simulink model "pdl_nonlinear_hw1"  (R2017a)
settings: Solver=VariableStepAuto  StartTime=0.0  StopTime=duration  RelTol=1e-3
values from neighbouring files (symbols this model uses):
  b = 0.1    [pendulum_hw1.m]
  f_p = 0    [pendulum_hw1.m]
  g = 9.81    [pendulum_hw1.m]
  k = 0.15    [pendulum_hw1.m]
  L = 1.4    [pendulum_hw1.m]
  m = 0.75    [pendulum_hw1.m]
  M = 1    [pendulum_hw1.m]
  Ts = 0.001    [pendulum_hw1.m]
  w_p = 0    [pendulum_hw1.m]
libraries: simulink x2
settings Model: Creator=Salmon  LastModifiedBy=Salmon

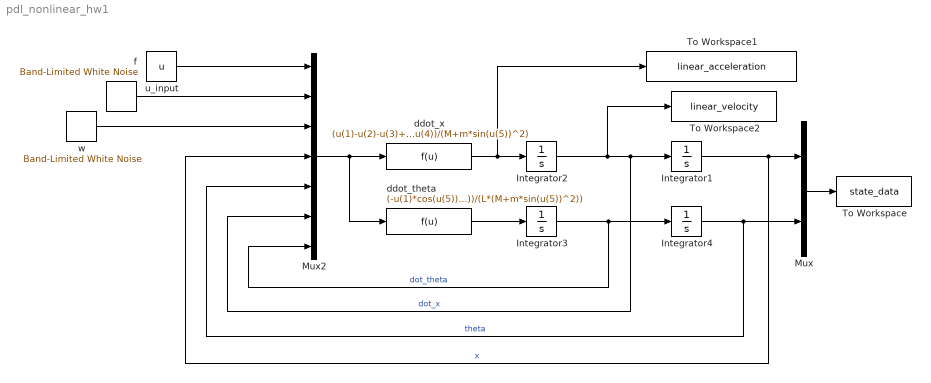
== system pdl_nonlinear_hw1 ==
  Integrator{1..4} (4 alike) : Integrator
  Mux : Mux  Inputs=2
  Mux2 : Mux  Inputs=7
  To Workspace : ToWorkspace  VariableName=state_data  SaveFormat=Structure With Time  SampleTime=-1
  To Workspace1 : ToWorkspace  VariableName=linear_acceleration  SaveFormat=Structure With Time  SampleTime=-1
  To Workspace2 : ToWorkspace  VariableName=linear_velocity  SaveFormat=Structure With Time  SampleTime=-1
  ddot_theta : Fcn  Expr=(-u(1)*cos(u(5))+u(3)*cos(u(5))-m*L*u(7)^2*sin(u(5))*cos(u(5))+(M+m)*g*sin(u(5))-(M/m)*u(2)*cos(u(5))+b*u(6)*cos(u(5))+k*u(4)*cos(u(5)))/(L*(M+m*sin(u(5))^2))
  ddot_x : Fcn  Expr=(u(1)-u(2)-u(3)+u(2)*cos(u(5))^2+m*L*u(7)^2*sin(u(5))-m*g*sin(u(5))*cos(u(5))-b*u(6)-k*u(4))/(M+m*sin(u(5))^2)
  f : simulink/Sources/Band-Limited White Noise  Cov=[f_p]  Ts=Ts  seed=[23341]
  u_input : Constant  Value=u
  w : simulink/Sources/Band-Limited White Noise  Cov=[w_p]  Ts=Ts  seed=[23341]
  wires:
  w/1 -> Mux2/3
  f/1 -> Mux2/2
  u_input/1 -> Mux2/1
  Mux2/1 -> ddot_theta/1, ddot_x/1
  ddot_x/1 -> To Workspace1/1, Integrator2/1
  Integrator2/1 -> To Workspace2/1, Mux2/6, Integrator1/1  "dot_x"
  ddot_theta/1 -> Integrator3/1
  Integrator3/1 -> Mux2/7, Integrator4/1  "dot_theta"
  Integrator1/1 -> Mux/1, Mux2/4  "x"
  Integrator4/1 -> Mux/2, Mux2/5  "theta"
  Mux/1 -> To Workspace/1
